simulink model "counter"  (Simulink 6.6)
settings: Solver=FixedStepDiscrete  StartTime=0.0  StopTime=10.0  FixedStep=1  RelTol=1e-3
settings Model: Creator=Nyenyec  LastModifiedBy=ksmyth

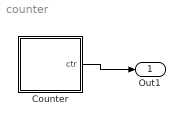
== system counter ==
  Counter : Stateflow chart
  Out1 : Outport
  wires:
  Counter/1(ctr) -> Out1/1

== stateflow chart Counter ==
  settings: executeAtInitialization=1
  state s1
  (default) -> s1
  s1 -> s1 [order 1] : [ctr < maxVal] / ctr = ctr+1;
  s1 -> s1 [order 2] : [ctr >= maxVal] / ctr = 0;
  data: ctr output double =1; maxVal constant double =4
